simulink model "Inner3_tmp"  (Simulink 8.3)
settings: Solver=FixedStepDiscrete  StartTime=0.0  StopTime=20  RelTol=1e-3
settings Model: Creator=scaife  LastModifiedBy=bourbouh  CovSFcnEnable=on  ExtModeAutoUpdateStatusClock=off
settings DataIOCC: SignalLoggingName=sigsOut
settings DebuggingCC: SaveWithParameterizedLinksMsg=none  SignalResolutionControl=TryResolveAllWithWarning  SolverPrmCheckMsg=none  MultiTaskDSMMsg=warning  MultiTaskCondExecSysMsg=none  FrameProcessingCompatibilityMsg=error  StateNameClashWarn=none
settings HardwareCC: TargetUnknown=on
settings SFSimCC: SimParseCustomCode=off

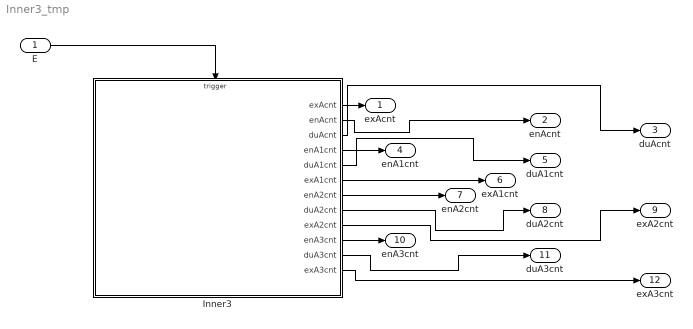
== system Inner3_tmp ==
  E : Inport
  Inner3 : Stateflow chart  TreatAsAtomicUnit=on
      settings: PermitHierarchicalResolution=ParametersOnly
  exAcnt : Outport
  enAcnt : Outport  Port=2
  duAcnt : Outport  Port=3
  enA1cnt : Outport  Port=4
  duA1cnt : Outport  Port=5
  exA1cnt : Outport  Port=6
  enA2cnt : Outport  Port=7
  duA2cnt : Outport  Port=8
  exA2cnt : Outport  Port=9
  enA3cnt : Outport  Port=10
  duA3cnt : Outport  Port=11
  exA3cnt : Outport  Port=12
  wires:
  E/1 -> Inner3/Trigger
  Inner3/1(exAcnt) -> exAcnt/1
  Inner3/2(enAcnt) -> enAcnt/1
  Inner3/3(duAcnt) -> duAcnt/1
  Inner3/4(enA1cnt) -> enA1cnt/1
  Inner3/5(duA1cnt) -> duA1cnt/1
  Inner3/6(exA1cnt) -> exA1cnt/1
  Inner3/7(enA2cnt) -> enA2cnt/1
  Inner3/8(duA2cnt) -> duA2cnt/1
  Inner3/9(exA2cnt) -> exA2cnt/1
  Inner3/12(exA3cnt) -> exA3cnt/1
  Inner3/10(enA3cnt) -> enA3cnt/1
  Inner3/11(duA3cnt) -> duA3cnt/1

== stateflow chart Inner3 ==
  state A/
    en: enAcnt++;
    du: duAcnt++;
    ex: exAcnt++;
    state A1/
      en: enA1cnt++;
      du: duA1cnt++;
      ex: exA1cnt++;
    state A2/
      en: enA2cnt++;
      du: duA2cnt++;
      ex: exA2cnt++;
    state A3/
      en: enA3cnt++;
      du: duA3cnt++;
      ex: exA3cnt++;
    A -> (junction 7) : E
    (junction 7) -> A1 [order 3] : [duAcnt%%3==0]
    (junction 7) -> A3 [order 1] : [duAcnt%%3==2]
    (junction 7) -> A2 [order 2] : [duAcnt%%3==1]
    (default) -> A1
  (default) -> A
  data: exAcnt output int32; enAcnt output int32; duAcnt output int32; enA1cnt output int32; duA1cnt output int32; exA1cnt output int32; enA2cnt output int32; duA2cnt output int32; exA2cnt output int32; enA3cnt output int32; duA3cnt output int32; exA3cnt output int32
  events: E input EITHER_EDGE_EVENT
